simulink model "trajectory_tracking_Taeyoung_Lee"  (R2020b)
settings: Solver=ode15s  StartTime=0.0  StopTime=10  RelTol=10e-9
settings Model: Creator=iketa  LastModifiedBy=kt012
settings DebuggingCC: ArithmeticOperatorsInVariantConditions=warning
settings SFSimCC: CustomCodeUndefinedFunction=UseInterfaceOnly

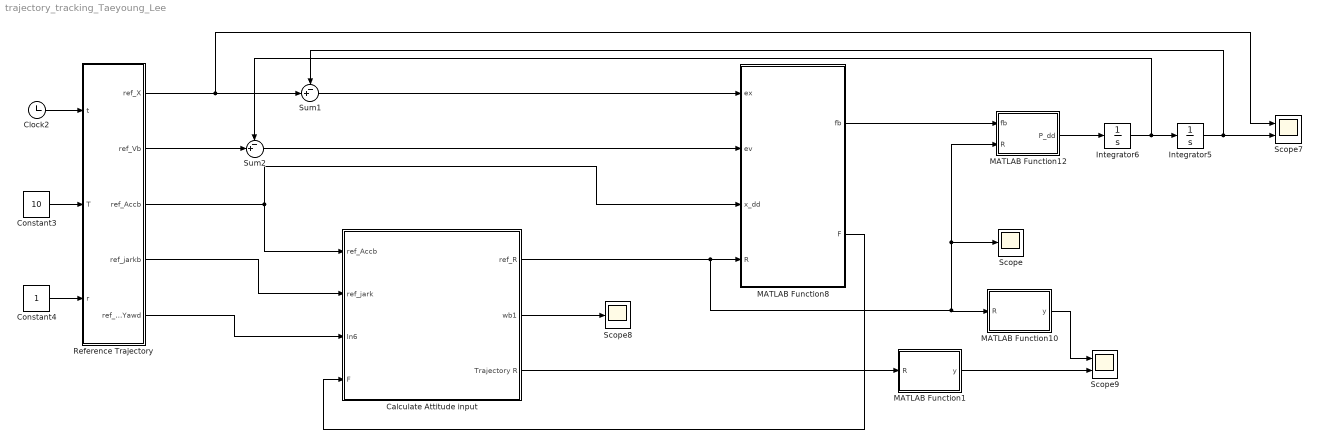
== system trajectory_tracking_Taeyoung_Lee ==
  Calculate Attitude input : Subsystem
  Clock2 : Clock
  Constant3 : Constant  Value=10
  Constant4 : Constant
  Integrator5 : Integrator  InitialCondition=[0;0;0]
  Integrator6 : Integrator  InitialCondition=[0;0;0]
  MATLAB Function1 : MATLAB Function  TreatAsAtomicUnit=on
  MATLAB Function10 : MATLAB Function  TreatAsAtomicUnit=on
  MATLAB Function12 : MATLAB Function  TreatAsAtomicUnit=on
  MATLAB Function8 : MATLAB Function
  Reference Trajectory : MATLAB Function  TreatAsAtomicUnit=on
  Scope : Scope
  Scope7 : Scope  NumInputPorts=2
  Scope8 : Scope
  Scope9 : Scope  NumInputPorts=2
  Sum1 : Sum  Inputs=-+|
  Sum2 : Sum  Inputs=-+|
  wires:
  Constant4/1 -> Reference Trajectory/3(r)
  Constant3/1 -> Reference Trajectory/2(T)
  Clock2/1 -> Reference Trajectory/1(t)
  Integrator5/1 -> Scope7/2, Sum1/1
  MATLAB Function8/1(fb) -> MATLAB Function12/1(fb)
  Integrator6/1 -> Sum2/1, Integrator5/1
  Reference Trajectory/3(ref_Accb) -> MATLAB Function8/3(x_dd), Calculate Attitude input/1(ref_Accb)
  Reference Trajectory/1(ref_X) -> Sum1/2, Scope7/1
  Reference Trajectory/2(ref_Vb) -> Sum2/2
  Sum1/1 -> MATLAB Function8/1(ex)
  Sum2/1 -> MATLAB Function8/2(ev)
  MATLAB Function12/1(P_dd) -> Integrator6/1
  MATLAB Function8/2(F) -> Calculate Attitude input/4(F)
  Reference Trajectory/4(ref_jarkb) -> Calculate Attitude input/2(ref_jark)
  Reference Trajectory/5(ref_Yaw_Yawd) -> Calculate Attitude input/3(In6)
  Calculate Attitude input/2(wb1) -> Scope8/1
  MATLAB Function10/1(y) -> Scope9/1
  Calculate Attitude input/1(ref_R) -> MATLAB Function12/2(R), Scope/1, MATLAB Function10/1(R), MATLAB Function8/4(R)
  Calculate Attitude input/3(Trajectory R) -> MATLAB Function1/1(R)
  MATLAB Function1/1(y) -> Scope9/2

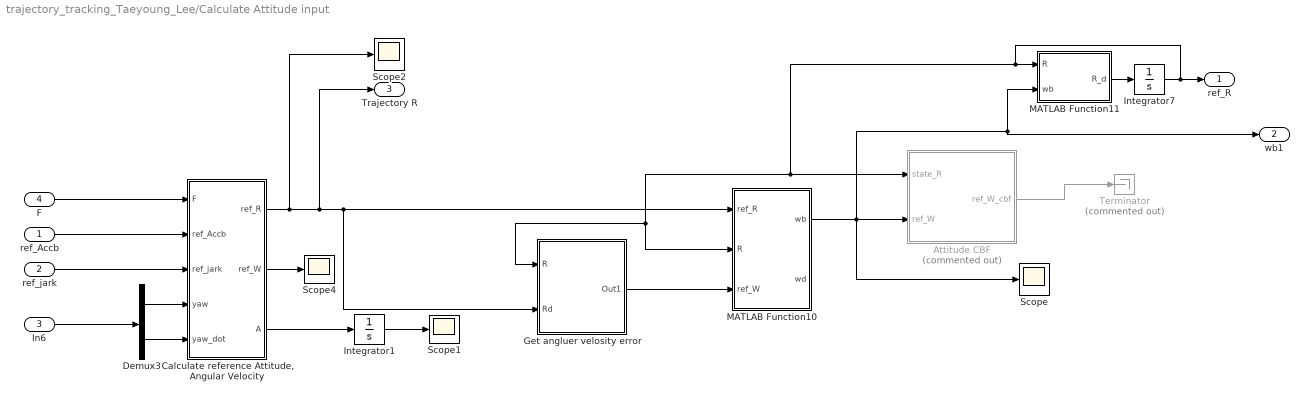
== system trajectory_tracking_Taeyoung_Lee/Calculate Attitude input ==
  ref_Accb : Inport
  ref_jark : Inport  Port=2
  In6 : Inport  Port=3
  F : Inport  Port=4
  Attitude CBF : MATLAB Function  Commented=on  TreatAsAtomicUnit=on
  "Calculate reference Attitude, Angular Velocity" : MATLAB Function  TreatAsAtomicUnit=on
  Demux3 : Demux  Outputs=2
  Get angluer velosity error : Subsystem
  Integrator1 : Integrator  InitialCondition=[0.8451 0 0.5347; -0.0864 0.9868 0.1366; -0.5276 -0.1616 0.8339]
  Integrator7 : Integrator  InitialCondition=[1 0 0; 0 1 0; 0 0 1]
  MATLAB Function10 : MATLAB Function  TreatAsAtomicUnit=on
  MATLAB Function11 : MATLAB Function  TreatAsAtomicUnit=on
  Scope{,1..2,4} (4 alike) : Scope
  Terminator : Terminator  Commented=on
  ref_R : Outport
  wb1 : Outport  Port=2
  Trajectory R : Outport  Port=3
  wires:
  "Calculate reference Attitude, Angular Velocity"/2(ref_W) -> Scope4/1
  Integrator7/1 -> Attitude CBF/1(state_R), MATLAB Function10/2(R), Get angluer velosity error/1(R), MATLAB Function11/1(R), ref_R/1
  F/1 -> "Calculate reference Attitude, Angular Velocity"/1(F)
  Demux3/1 -> "Calculate reference Attitude, Angular Velocity"/4(yaw)
  "Calculate reference Attitude, Angular Velocity"/1(ref_R) -> Scope2/1, Get angluer velosity error/2(Rd), MATLAB Function10/1(ref_R), Trajectory R/1
  MATLAB Function11/1(R_d) -> Integrator7/1
  Demux3/2 -> "Calculate reference Attitude, Angular Velocity"/5(yaw_dot)
  ref_Accb/1 -> "Calculate reference Attitude, Angular Velocity"/2(ref_Accb)
  In6/1 -> Demux3/1
  ref_jark/1 -> "Calculate reference Attitude, Angular Velocity"/3(ref_jark)
  Attitude CBF/1(ref_W_cbf) -> Terminator/1
  Integrator1/1 -> Scope1/1
  "Calculate reference Attitude, Angular Velocity"/3(A) -> Integrator1/1
  MATLAB Function10/1(wb) -> wb1/1, MATLAB Function11/2(wb), Attitude CBF/2(ref_W), Scope/1
  Get angluer velosity error/1(Out1) -> MATLAB Function10/3(ref_W)

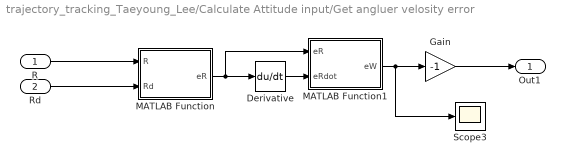
== system trajectory_tracking_Taeyoung_Lee/Calculate Attitude input/Get angluer velosity error ==
  R : Inport
  Rd : Inport  Port=2
  Derivative : Derivative
  Gain : Gain  Gain=-1
  MATLAB Function : MATLAB Function  TreatAsAtomicUnit=on
  MATLAB Function1 : MATLAB Function  TreatAsAtomicUnit=on
  Scope3 : Scope
  Out1 : Outport
  wires:
  R/1 -> MATLAB Function/1(R)
  MATLAB Function/1(eR) -> MATLAB Function1/1(eR), Derivative/1
  MATLAB Function1/1(eW) -> Scope3/1, Gain/1
  Gain/1 -> Out1/1
  Derivative/1 -> MATLAB Function1/2(eRdot)
  Rd/1 -> MATLAB Function/2(Rd)

== matlab function trajectory_tracking_Taeyoung_Lee/Reference Trajectory ==
  data: ref_X output; ref_Vb output; ref_Accb output; ref_jarkb output; t input; T input; r input; ref_Yaw_Yawd output
function [ref_X, ref_Vb, ref_Accb, ref_jarkb, ref_Yaw_Yawd] = fcn(t,T,r)
% 軌道生成
w = 2 * pi/T;          % 角周波数

% 中心　半径　　
c = [0;0;0];

ref_X = c + r*[sin(w*t); cos(w*t); 0];
ref_Vb = r*[w*cos(w*t); -w*sin(w*t); 0];
ref_Accb = [-r*w^2*sin(w*t); -r*w^2*cos(w*t); 9.8];
ref_jarkb = r*[-w^3*cos(w*t); w^3*sin(w*t); 0];
ref_Yaw_Yawd = [0, 0]';

== matlab function trajectory_tracking_Taeyoung_Lee/MATLAB Function10 ==
  data: R input; y output
function y = fcn(R)
Rtranspose = R';
eR = (R - Rtranspose)/2;

y = [eR(3, 2) -eR(3, 1) eR(2, 1)]';

== matlab function trajectory_tracking_Taeyoung_Lee/MATLAB Function1 ==
  data: R input; y output
function y = fcn(R)
Rtranspose = R';
eR = (R - Rtranspose)/2;

y = [eR(3, 2) -eR(3, 1) eR(2, 1)]';

== matlab function trajectory_tracking_Taeyoung_Lee/Calculate Attitude input/Get angluer velosity error/MATLAB Function ==
  data: R input; eR output; Rd input
function eR = fcn(R, Rd)
R = eye(3);
eR = Rd'*R;

== matlab function trajectory_tracking_Taeyoung_Lee/Calculate Attitude input/Get angluer velosity error/MATLAB Function1 ==
  data: eR input; eW output; eRdot input
function eW = fcn(eR, eRdot)

tmp= pinv(eR) * eRdot;
eW = [tmp(3, 2) tmp(1, 3) tmp(2, 1)]';

== matlab function trajectory_tracking_Taeyoung_Lee/Calculate Attitude input/Calculate reference Attitude, Angular Velocity ==
  data: ref_R output; ref_W output; F input; ref_Accb input; ref_jark input; yaw input; yaw_dot input; A output
function [ref_R,ref_W,A]= fcn(F, ref_Accb, ref_jark, yaw, yaw_dot)

% Flat Outputから内部状態と入力揚力を計算

m = 0.03;
F = F;
Xc = [cos(yaw) sin(yaw) 0]';          % よー角のベクトル　Rc(3)
Yc = [-sin(yaw) cos(yaw) 0]';
dXc = yaw_dot * Yc; % よー角のベクトルの微分
dYc = -yaw_dot * Xc; 

% 所望の姿勢を計算している
% 軌道の加速度のベクトル: b3 を計算
Zb = F / norm(F);   
%
% Xb = cross(Yc, Zb)/norm(cross(Yc, Zb));
% Yb = cross(Zb, Xb); 
Yb = cross(Zb,Xc)/norm(cross(Zb,Xc));
Xb = cross(Yb,Zb);
ref_R = [Xb Yb Zb] ;

% 加加速度ベクトルを計算
dfZb = ref_jark;
  
% 目標の姿勢のz軸方向のベクトルの微分を計算
dZb = dfZb/norm(F) - F * dot(F, dfZb)/norm(F)^3; % Zb_dot---------- dot(　fb1/norm(fb1) )

% 目標の姿勢のx軸方向のベクトルを計算
dnorm_Zb_Xc2 = norm(cross(dYc, Zb) + cross(Yc, dZb));
dXb = (cross(dYc, Zb) + cross(Yc, dZb))/dnorm_Zb_Xc2 - cross(Yc, Zb) * dot(cross(Yc, Zb),( cross(dYc, Zb) + cross(Yc, dZb)))/dnorm_Zb_Xc2^3;
   
% 目標の姿勢のy軸方向のベクトルを計算
dYb = cross(dZb, Xb) + cross(Zb, dXb) ;  %dot_b2 = dotb3とb1 の外積と　b3とdot_b1の外積　の和　--------- dot(cross(b3, b1))


% wy = dot(Xb, ref_jark) / dot(Zb, ref_Accb);
% wx = - dot(Yb, ref_jark) / dot(Zb, ref_Accb);
wy = dot(Xb, ref_jark) / dot(Zb, F);
wx = - dot(Yb, ref_jark) / dot(Zb, F);
wz = (yaw_dot * dot(Xc, Xb) + wy * dot(Yc, Zb))/norm(cross(Yc, Zb));
ref_W = [wx wy wz];
ref_wd = [0,-wz,wy; wz,0,-wx; -wy,wx,0];
A =ref_R *ref_wd;

== matlab function trajectory_tracking_Taeyoung_Lee/MATLAB Function8 ==
  data: ex input; fb output; ev input; x_dd input; R input; F output
function [fb, F]= fcn(ex,ev,x_dd,R)
m = 1.0;
e3 = [0;0;1];

kx_x = 2.0;
kx_y = 2.0;
kx_z = 3;

kv_x = 10;
kv_y = 6;
kv_z = 50;

ex_x = kx_x*ex(1);
ex_y = kx_y*ex(2);
ex_z = kx_z*ex(3);
ex_d = [ex_x; ex_y; ex_z];

ev_x = kv_x*ev(1);
ev_y = kv_y*ev(2);
ev_z = kv_z*ev(3);
ev_d = [ev_x; ev_y; ev_z];
 
u = dot(ex_d + ev_d + m*x_dd, R*e3);
F = ex_d + ev_d + m*x_dd;

fb = u;

== matlab function trajectory_tracking_Taeyoung_Lee/Calculate Attitude input/MATLAB Function10 ==
  data: ref_R input; R input; wb output; ref_W input; wd output
function [wb, wd]= fcn(ref_R,R,ref_W)
R_T = R';
Rd_T = ref_R';
eR = (Rd_T*R - R_T*ref_R)/2;

kR = 1.0;
wx = ref_W(1);
wy = ref_W(2);
wz = ref_W(3);
wd = [0 -wz wy; wz 0 -wx;-wy wx 0];
u = -kR * eR + wd;

wb = u;

== matlab function trajectory_tracking_Taeyoung_Lee/Calculate Attitude input/MATLAB Function11 ==
  data: R input; wb input; R_d output
function R_d = fcn(R,wb)
u = R * wb;
R_d = u;

== matlab function trajectory_tracking_Taeyoung_Lee/MATLAB Function12 ==
  data: fb input; P_dd output; R input
function P_dd = fcn(fb,R)
e3 = [0;0;1];
g = 9.8;
m = 1.0;

u = (fb*R*e3/m) - g*e3 ;

P_dd = u;

== matlab function trajectory_tracking_Taeyoung_Lee/Calculate Attitude input/Attitude CBF ==
  data: state_R input; ref_W input; ref_W_cbf output
function ref_W_cbf = fcn(state_R, ref_W)
ref_W = [ref_W(3, 2), -ref_W(3, 1), ref_W(2, 1)];
theta = 0.1;
coder.extrinsic('quadprog')
tmp = zeros(3, 1);
e3 = [0; 0; 1];
e3_wedge = [0 -1 0; 1 0 0; 0 0 0];
H = eye(3);
f = -2*ref_W;
% ref_W
A = e3'*state_R*e3_wedge;
B = (e3'*state_R*e3 - cos(theta));



tmp  = quadprog(H, f, A, B);
ref_W_cbf = [0      -tmp(3)   tmp(2); 
             tmp(3)  0       -tmp(1); 
             -tmp(2) tmp(1)   0];
if A * tmp > B
    A * tmp
    B
end
